simulink model "microgrid_healthy_load_profiling_DDR_revF"  (Simulink 7.9)
settings: Solver=ode3  SolverMode=SingleTasking  StartTime=0.0  StopTime=12  FixedStep=5*10^(-5)  RelTol=1e-3
undefined symbols (not defined in the file): D1, Delta, tl1, tl2, tl3, tl4, tl5, tl6, Ts
libraries: powerlib x108, powerlib_extras x36
(part 2 of 2)

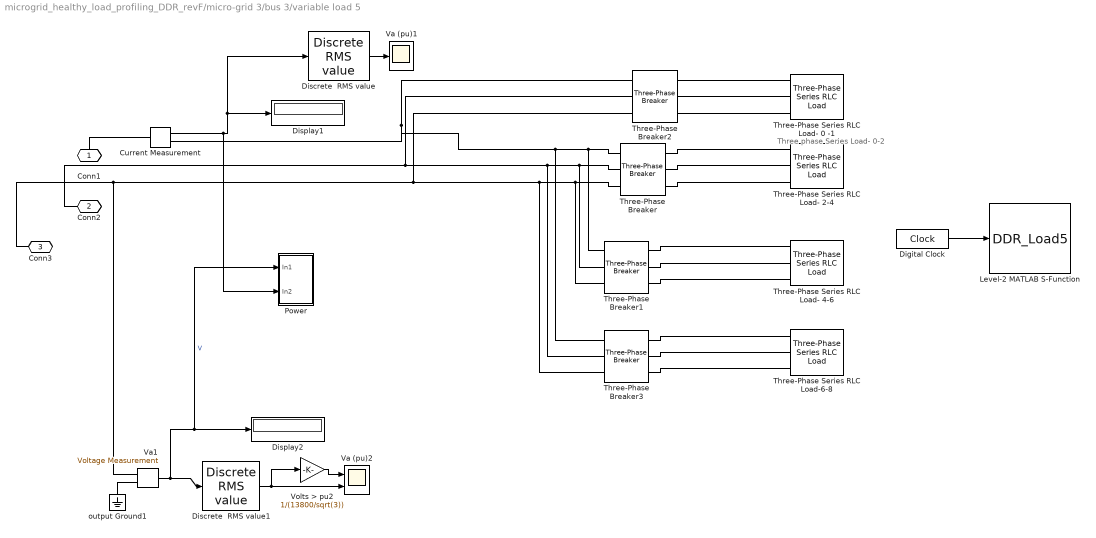
== system microgrid_healthy_load_profiling_DDR_revF/micro-grid 3/bus 3/variable load 5 ==
  note: Three phase Series Load- 0-2
  Current Measurement : powerlib/Measurements/Current Measurement  PhasorSimulation=off  OutputType=Complex  PSBequivalent=0
  Digital Clock : DigitalClock  SampleTime=Ts
  Discrete  RMS value : powerlib_extras/Discrete Measurements/Discrete  RMS value  Freq=60  Mag_Init=0  Ts=Ts
  Discrete  RMS value1 : powerlib_extras/Discrete Measurements/Discrete  RMS value  Freq=60  Mag_Init=0  Ts=Ts
  Display1 : Display
  Display2 : Display
  Level-2 MATLAB S-Function : M-S-Function  FunctionName=DDR_Load5  Parameters=tl5
  Power : Subsystem
  Three-Phase Series RLC Load- 0 -1 : powerlib/Elements/Three-Phase Series RLC Load  LConnTagsString=A|B|C  Configuration=Y (grounded)  NominalVoltage=13800  NominalFrequency=60  ActivePower=1.6e6  InductivePower=1.92e6  CapacitivePower=0  Measurements=None  LoadType=constant Z
  Three-Phase Series RLC Load- 2-4 : powerlib/Elements/Three-Phase Series RLC Load  LConnTagsString=A|B|C  Configuration=Y (grounded)  NominalVoltage=13800  NominalFrequency=60  ActivePower=2e6  InductivePower=0  CapacitivePower=1.5e6  Measurements=None  LoadType=constant Z
  Three-Phase Series RLC Load- 4-6 : powerlib/Elements/Three-Phase Series RLC Load  LConnTagsString=A|B|C  Configuration=Y (grounded)  NominalVoltage=13800  NominalFrequency=60  ActivePower=1.85e6  InductivePower=1.68e6  CapacitivePower=0  Measurements=None  LoadType=constant Z
  Three-Phase Series RLC Load-6-8 : powerlib/Elements/Three-Phase Series RLC Load  LConnTagsString=A|B|C  Configuration=Y (grounded)  NominalVoltage=13800  NominalFrequency=60  ActivePower=1.55e6  InductivePower=1.96e6  CapacitivePower=0  Measurements=None  LoadType=constant Z
  Three-Phase Breaker : powerlib/Elements/Three-Phase Breaker  InitialState=open  SwitchA=on  SwitchB=on  SwitchC=on  SwitchTimes=[tl5(1)/60 tl5(2)/60]  External=off  BreakerResistance=0.001  SnubberResistance=1e6  SnubberCapacitance=inf  Measurements=None
  Three-Phase Breaker1 : powerlib/Elements/Three-Phase Breaker  InitialState=open  SwitchA=on  SwitchB=on  SwitchC=on  SwitchTimes="[tl5(2)/60  tl5(3)/60]"  External=off  BreakerResistance=0.001  SnubberResistance=1e6  SnubberCapacitance=inf  Measurements=None
  Three-Phase Breaker2 : powerlib/Elements/Three-Phase Breaker  InitialState=closed  SwitchA=on  SwitchB=on  SwitchC=on  SwitchTimes=[tl5(1)/60]  External=off  BreakerResistance=0.001  SnubberResistance=1e6  SnubberCapacitance=inf  Measurements=None
  Three-Phase Breaker3 : powerlib/Elements/Three-Phase Breaker  InitialState=open  SwitchA=on  SwitchB=on  SwitchC=on  SwitchTimes=[tl5(3)/60]  External=off  BreakerResistance=0.001  SnubberResistance=1e6  SnubberCapacitance=inf  Measurements=None
  Va (pu)1 : Scope
      settings: TickLabels=on  TimeRange=2  YMin=-0.8  YMax=0.8  SaveName=vf6
  Va (pu)2 : Scope  NumInputPorts=2
      settings: TickLabels=on  TimeRange=3  YMin=0.8979~7153.5  YMax=0.8991~7163.5  SaveName=vf2
  Va1 : powerlib/Measurements/Voltage Measurement  Tag=PoWeRsYsTeMmEaSuReMeNt  PhasorSimulation=off  OutputType=Magnitude  PSBequivalent=0
  Volts > pu2 : Gain  Gain=1/(13800/sqrt(3))  SaturateOnIntegerOverflow=on  OutDataTypeStr=Inherit: Same as input  ParamDataTypeStr=Inherit: Same as input
  output Ground1 : powerlib/Elements/Ground  LConnTagsString=a
  Conn1 : PMIOPort  Port=1  Side=Left
  Conn2 : PMIOPort  Port=2  Side=Left
  Conn3 : PMIOPort  Port=3  Side=Left
  wires:
  Va1/1 -> Display2/1, Power/1(In1), Discrete  RMS value1/1  "V"
  Current Measurement/1 -> Display1/1, Discrete  RMS value/1, Power/2(In2)
  Discrete  RMS value/1 -> Va (pu)1/1
  Discrete  RMS value1/1 -> Va (pu)2/2, Volts > pu2/1
  Volts > pu2/1 -> Va (pu)2/1
  Digital Clock/1 -> Level-2 MATLAB S-Function/1
  connections:
  Three-Phase Breaker/RConn1 -- Three-Phase Series RLC Load- 2-4/LConn1
  Three-Phase Breaker/RConn2 -- Three-Phase Series RLC Load- 2-4/LConn2
  Three-Phase Breaker/RConn3 -- Three-Phase Series RLC Load- 2-4/LConn3
  Three-Phase Breaker1/RConn1 -- Three-Phase Series RLC Load- 4-6/LConn1
  Three-Phase Breaker1/RConn2 -- Three-Phase Series RLC Load- 4-6/LConn2
  Three-Phase Breaker1/RConn3 -- Three-Phase Series RLC Load- 4-6/LConn3
  Three-Phase Breaker2/LConn1 -- Three-Phase Breaker/LConn1 -- Three-Phase Breaker1/LConn1 -- Three-Phase Breaker3/LConn1 -- Current Measurement/RConn1
  Three-Phase Breaker2/LConn2 -- Three-Phase Breaker/LConn2 -- Three-Phase Breaker1/LConn2 -- Three-Phase Breaker3/LConn2 -- Conn2/RConn1
  Conn3/RConn1 -- Va1/LConn1 -- Three-Phase Breaker2/LConn3 -- Three-Phase Breaker/LConn3 -- Three-Phase Breaker1/LConn3 -- Three-Phase Breaker3/LConn3
  Three-Phase Breaker2/RConn2 -- Three-Phase Series RLC Load- 0 -1/LConn2
  Three-Phase Breaker2/RConn3 -- Three-Phase Series RLC Load- 0 -1/LConn3
  output Ground1/LConn1 -- Va1/LConn2
  Conn1/RConn1 -- Current Measurement/LConn1
  Three-Phase Breaker2/RConn1 -- Three-Phase Series RLC Load- 0 -1/LConn1
  Three-Phase Breaker3/RConn1 -- Three-Phase Series RLC Load-6-8/LConn1
  Three-Phase Breaker3/RConn2 -- Three-Phase Series RLC Load-6-8/LConn2
  Three-Phase Breaker3/RConn3 -- Three-Phase Series RLC Load-6-8/LConn3

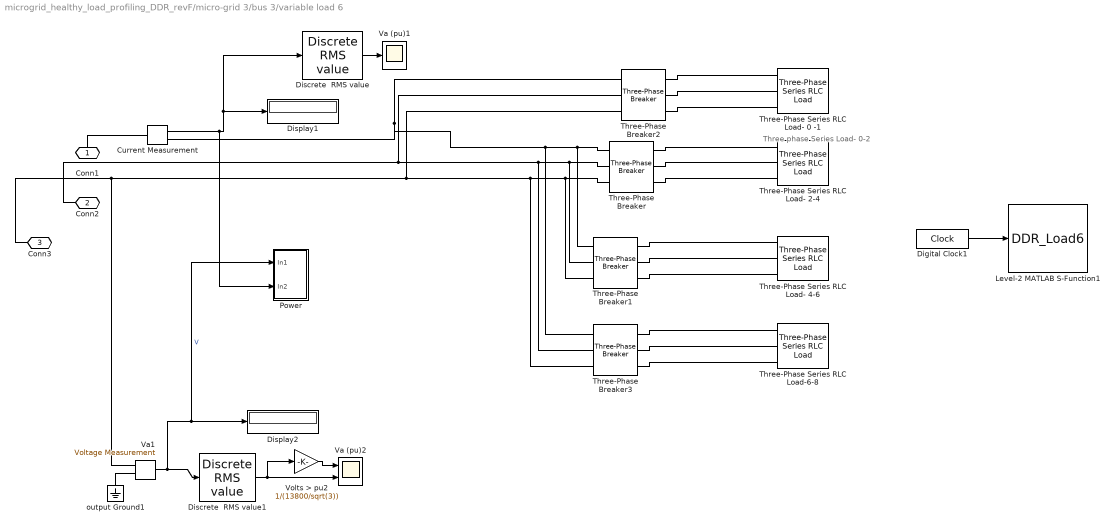
== system microgrid_healthy_load_profiling_DDR_revF/micro-grid 3/bus 3/variable load 6 ==
  note: Three phase Series Load- 0-2
  Current Measurement : powerlib/Measurements/Current Measurement  PhasorSimulation=off  OutputType=Complex  PSBequivalent=0
  Digital Clock1 : DigitalClock  SampleTime=Ts
  Discrete  RMS value : powerlib_extras/Discrete Measurements/Discrete  RMS value  Freq=60  Mag_Init=0  Ts=Ts
  Discrete  RMS value1 : powerlib_extras/Discrete Measurements/Discrete  RMS value  Freq=60  Mag_Init=0  Ts=Ts
  Display1 : Display
  Display2 : Display
  Level-2 MATLAB S-Function1 : M-S-Function  FunctionName=DDR_Load6  Parameters=tl6
  Power : Subsystem
  Three-Phase Series RLC Load- 0 -1 : powerlib/Elements/Three-Phase Series RLC Load  LConnTagsString=A|B|C  Configuration=Y (grounded)  NominalVoltage=13800  NominalFrequency=60  ActivePower=1.7e6  InductivePower=1.83e6  CapacitivePower=0  Measurements=None  LoadType=constant Z
  Three-Phase Series RLC Load- 2-4 : powerlib/Elements/Three-Phase Series RLC Load  LConnTagsString=A|B|C  Configuration=Y (grounded)  NominalVoltage=13800  NominalFrequency=60  ActivePower=2e6  InductivePower=0  CapacitivePower=1.5e6  Measurements=None  LoadType=constant Z
  Three-Phase Series RLC Load- 4-6 : powerlib/Elements/Three-Phase Series RLC Load  LConnTagsString=A|B|C  Configuration=Y (grounded)  NominalVoltage=13800  NominalFrequency=60  ActivePower=2.1e6  InductivePower=1.356e6  CapacitivePower=0  Measurements=None  LoadType=constant Z
  Three-Phase Series RLC Load-6-8 : powerlib/Elements/Three-Phase Series RLC Load  LConnTagsString=A|B|C  Configuration=Y (grounded)  NominalVoltage=13800  NominalFrequency=60  ActivePower=1.6e6  InductivePower=1.92e6  CapacitivePower=0  Measurements=None  LoadType=constant Z
  Three-Phase Breaker : powerlib/Elements/Three-Phase Breaker  InitialState=open  SwitchA=on  SwitchB=on  SwitchC=on  SwitchTimes=[tl6(1)/60 tl6(2)/60]  External=off  BreakerResistance=0.001  SnubberResistance=1e6  SnubberCapacitance=inf  Measurements=None
  Three-Phase Breaker1 : powerlib/Elements/Three-Phase Breaker  InitialState=open  SwitchA=on  SwitchB=on  SwitchC=on  SwitchTimes="[tl6(2)/60  tl6(3)/60]"  External=off  BreakerResistance=0.001  SnubberResistance=1e6  SnubberCapacitance=inf  Measurements=None
  Three-Phase Breaker2 : powerlib/Elements/Three-Phase Breaker  InitialState=closed  SwitchA=on  SwitchB=on  SwitchC=on  SwitchTimes=[tl6(1)/60]  External=off  BreakerResistance=0.001  SnubberResistance=1e6  SnubberCapacitance=inf  Measurements=None
  Three-Phase Breaker3 : powerlib/Elements/Three-Phase Breaker  InitialState=open  SwitchA=on  SwitchB=on  SwitchC=on  SwitchTimes=[tl6(3)/60]  External=off  BreakerResistance=0.001  SnubberResistance=1e6  SnubberCapacitance=inf  Measurements=None
  Va (pu)1 : Scope
      settings: TickLabels=on  TimeRange=2  YMin=-0.8  YMax=0.8  SaveName=vf6
  Va (pu)2 : Scope  NumInputPorts=2
      settings: TickLabels=on  TimeRange=3  YMin=0.8979~7153.5  YMax=0.8991~7163.5  SaveName=vf2
  Va1 : powerlib/Measurements/Voltage Measurement  Tag=PoWeRsYsTeMmEaSuReMeNt  PhasorSimulation=off  OutputType=Magnitude  PSBequivalent=0
  Volts > pu2 : Gain  Gain=1/(13800/sqrt(3))  SaturateOnIntegerOverflow=on  OutDataTypeStr=Inherit: Same as input  ParamDataTypeStr=Inherit: Same as input
  output Ground1 : powerlib/Elements/Ground  LConnTagsString=a
  Conn1 : PMIOPort  Port=1  Side=Left
  Conn2 : PMIOPort  Port=2  Side=Left
  Conn3 : PMIOPort  Port=3  Side=Left
  wires:
  Volts > pu2/1 -> Va (pu)2/1
  Discrete  RMS value1/1 -> Volts > pu2/1, Va (pu)2/2
  Discrete  RMS value/1 -> Va (pu)1/1
  Current Measurement/1 -> Power/2(In2), Display1/1, Discrete  RMS value/1
  Va1/1 -> Discrete  RMS value1/1, Power/1(In1), Display2/1  "V"
  Digital Clock1/1 -> Level-2 MATLAB S-Function1/1
  connections:
  Three-Phase Breaker3/RConn3 -- Three-Phase Series RLC Load-6-8/LConn3
  Three-Phase Breaker3/RConn2 -- Three-Phase Series RLC Load-6-8/LConn2
  Three-Phase Breaker3/RConn1 -- Three-Phase Series RLC Load-6-8/LConn1
  Conn1/RConn1 -- Current Measurement/LConn1
  output Ground1/LConn1 -- Va1/LConn2
  Three-Phase Breaker1/LConn3 -- Three-Phase Breaker/LConn3 -- Three-Phase Breaker2/LConn3 -- Va1/LConn1 -- Conn3/RConn1 -- Three-Phase Breaker3/LConn3
  Three-Phase Breaker1/LConn2 -- Three-Phase Breaker/LConn2 -- Three-Phase Breaker2/LConn2 -- Conn2/RConn1 -- Three-Phase Breaker3/LConn2
  Three-Phase Breaker1/LConn1 -- Three-Phase Breaker/LConn1 -- Three-Phase Breaker2/LConn1 -- Current Measurement/RConn1 -- Three-Phase Breaker3/LConn1
  Three-Phase Breaker1/RConn3 -- Three-Phase Series RLC Load- 4-6/LConn3
  Three-Phase Breaker1/RConn2 -- Three-Phase Series RLC Load- 4-6/LConn2
  Three-Phase Breaker1/RConn1 -- Three-Phase Series RLC Load- 4-6/LConn1
  Three-Phase Breaker/RConn3 -- Three-Phase Series RLC Load- 2-4/LConn3
  Three-Phase Breaker/RConn2 -- Three-Phase Series RLC Load- 2-4/LConn2
  Three-Phase Breaker/RConn1 -- Three-Phase Series RLC Load- 2-4/LConn1
  Three-Phase Breaker2/RConn1 -- Three-Phase Series RLC Load- 0 -1/LConn1
  Three-Phase Breaker2/RConn3 -- Three-Phase Series RLC Load- 0 -1/LConn3
  Three-Phase Breaker2/RConn2 -- Three-Phase Series RLC Load- 0 -1/LConn2

== system microgrid_healthy_load_profiling_DDR_revF/microgrid-1/variable load 1/Power ==
  In1 : Inport
  In2 : Inport  Port=2
  Active & Reactive Power : powerlib_extras/Measurements/Active & Reactive Power  f1=60
  Add : Sum
  Demux : Demux  Outputs=2
  Math Function : Math  Operator=square  OutputSignalType=real  SaturateOnIntegerOverflow=on
  Math Function1 : Math  Operator=square  OutputSignalType=real  SaturateOnIntegerOverflow=on
  Sqrt : Sqrt  SaturateOnIntegerOverflow=on
  Va (pu)3 : Scope  NumInputPorts=2
      settings: TickLabels=on  TimeRange=2  YMin=206676~-125000  YMax=206700~175000  SaveName=vf3
  wires:
  Active & Reactive Power/1 -> Demux/1, Va (pu)3/2
  Demux/1 -> Math Function/1
  Math Function/1 -> Add/1
  Demux/2 -> Math Function1/1
  Math Function1/1 -> Add/2
  Add/1 -> Sqrt/1
  Sqrt/1 -> Va (pu)3/1
  In1/1 -> Active & Reactive Power/1
  In2/1 -> Active & Reactive Power/2

== system microgrid_healthy_load_profiling_DDR_revF/microgrid-1/variable load 2/Power ==
  In1 : Inport
  In2 : Inport  Port=2
  Active & Reactive Power : powerlib_extras/Measurements/Active & Reactive Power  f1=60
  Add : Sum
  Demux : Demux  Outputs=2
  Math Function : Math  Operator=square  OutputSignalType=real  SaturateOnIntegerOverflow=on
  Math Function1 : Math  Operator=square  OutputSignalType=real  SaturateOnIntegerOverflow=on
  Sqrt : Sqrt  SaturateOnIntegerOverflow=on
  Va (pu)3 : Scope  NumInputPorts=2
      settings: TickLabels=on  TimeRange=2  YMin=206676~-125000  YMax=206700~175000  SaveName=vf3
  wires:
  In2/1 -> Active & Reactive Power/2
  In1/1 -> Active & Reactive Power/1
  Sqrt/1 -> Va (pu)3/1
  Add/1 -> Sqrt/1
  Math Function1/1 -> Add/2
  Demux/2 -> Math Function1/1
  Math Function/1 -> Add/1
  Demux/1 -> Math Function/1
  Active & Reactive Power/1 -> Va (pu)3/2, Demux/1

== system microgrid_healthy_load_profiling_DDR_revF/micro-grid 3/bus 3/variable load 5/Power ==
  In1 : Inport
  In2 : Inport  Port=2
  Active & Reactive Power : powerlib_extras/Measurements/Active & Reactive Power  f1=60
  Add : Sum
  Demux : Demux  Outputs=2
  Math Function : Math  Operator=square  OutputSignalType=real  SaturateOnIntegerOverflow=on
  Math Function1 : Math  Operator=square  OutputSignalType=real  SaturateOnIntegerOverflow=on
  Sqrt : Sqrt  SaturateOnIntegerOverflow=on
  Va (pu)3 : Scope  NumInputPorts=2
      settings: TickLabels=on  TimeRange=2  YMin=206676~-125000  YMax=206700~175000  SaveName=vf3
  wires:
  Active & Reactive Power/1 -> Demux/1, Va (pu)3/2
  Demux/1 -> Math Function/1
  Math Function/1 -> Add/1
  Demux/2 -> Math Function1/1
  Math Function1/1 -> Add/2
  Add/1 -> Sqrt/1
  Sqrt/1 -> Va (pu)3/1
  In1/1 -> Active & Reactive Power/1
  In2/1 -> Active & Reactive Power/2

== system microgrid_healthy_load_profiling_DDR_revF/micro-grid 3/bus 3/variable load 6/Power ==
  In1 : Inport
  In2 : Inport  Port=2
  Active & Reactive Power : powerlib_extras/Measurements/Active & Reactive Power  f1=60
  Add : Sum
  Demux : Demux  Outputs=2
  Math Function : Math  Operator=square  OutputSignalType=real  SaturateOnIntegerOverflow=on
  Math Function1 : Math  Operator=square  OutputSignalType=real  SaturateOnIntegerOverflow=on
  Sqrt : Sqrt  SaturateOnIntegerOverflow=on
  Va (pu)3 : Scope  NumInputPorts=2
      settings: TickLabels=on  TimeRange=2  YMin=206676~-125000  YMax=206700~175000  SaveName=vf3
  wires:
  In2/1 -> Active & Reactive Power/2
  In1/1 -> Active & Reactive Power/1
  Sqrt/1 -> Va (pu)3/1
  Add/1 -> Sqrt/1
  Math Function1/1 -> Add/2
  Demux/2 -> Math Function1/1
  Math Function/1 -> Add/1
  Demux/1 -> Math Function/1
  Active & Reactive Power/1 -> Va (pu)3/2, Demux/1
